simulink model "bpsk_transmitter"  (R2020a)
settings: Solver=VariableStepAuto  StartTime=0.0  StopTime=200/100e3  RelTol=1e-3
PreLoadFcn:
  | setup_bpsk_transmitter
InitFcn:
  | setup_bpsk_transmitter
undefined symbols (not defined in the file): AXI4, Lite, tx_data, xlfda_numerator
libraries: xbsIndex_r4 x43, hdlsllib x4, simulink x1
settings Model: Creator=David Northcote  LastModifiedBy=david
settings SFSimCC: CustomCodeUndefinedFunction=UseInterfaceOnly

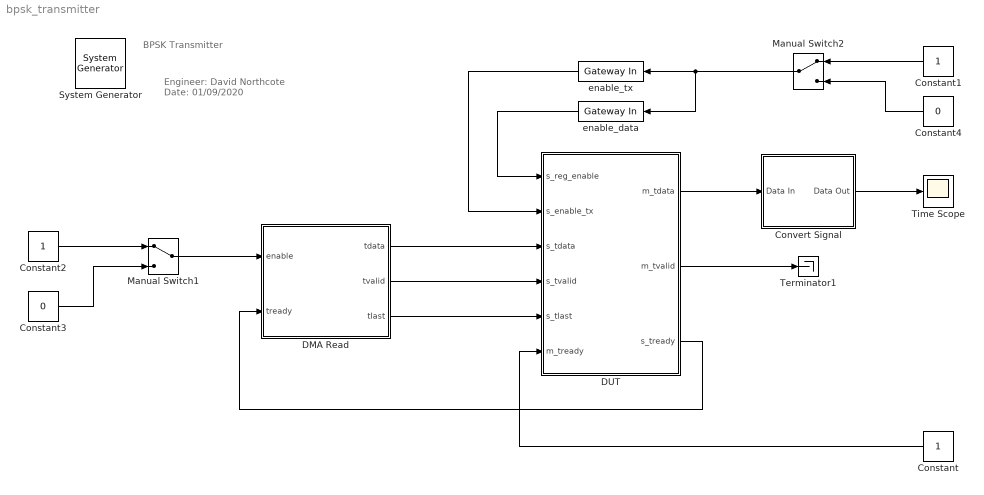
== system bpsk_transmitter ==
  note: Engineer:	David Northcote
      | Date:		01/09/2020
  note: BPSK Transmitter
  " System Generator" : xbsIndex_r4/ System Generator  Tag=genX  xilinxfamily=zynquplusRFSOC  part=xczu28dr  speed=-2-e  package=ffvg1517  synthesis_tool=Vivado  clock_wrapper=Clock Enables  directory=./netlist  proj_type=Vivado  Synth_file=Vivado Synthesis Defaults  Impl_file=Vivado Implementation Defaults  testbench=off  simulink_period=1/128e6  sysclk_period=(1/128e6)*1e9  dcm_input_clock_period=10  incr_netlist=off  trim_vbits=Everywhere in SubSystem  dbl_ovrd=According to Block Masks  core_generation=According to Block Masks  run_coregen=off  deprecated_control=off  eval_field=0  block_type=sysgen
  Constant : Constant  SampleTime=1/128e6
  Constant1 : Constant  OutDataTypeStr=boolean  SampleTime=1/(100e3)
  Constant2 : Constant  OutDataTypeStr=boolean  SampleTime=1/128e6
  Constant3 : Constant  Value=0  OutDataTypeStr=boolean  SampleTime=1/128e6
  Constant4 : Constant  Value=0  OutDataTypeStr=boolean  SampleTime=1/(100e3)
  Convert Signal : Subsystem
  DMA Read : Subsystem
  DUT : Subsystem
  Manual Switch1 : ManualSwitch
  Manual Switch2 : ManualSwitch
  Terminator1 : Terminator
  Time Scope : Scope
  enable_data : xbsIndex_r4/Gateway In  gui_display_data_type=Boolean  arith_type=Boolean  n_bits=16  bin_pt=14  preci_type=Single  exp_width=8  frac_width=24  rows=1  columns=1  quantization="Round  (unbiased: +/- Inf)"  overflow=Saturate  period=1/(100e3)  UseAsADC=off  ADCChannel='1'  interface=AXI4-Lite  automatic_assignment=off  address_offset=0  intf_name=''  intf_description=''  default_value=0  timing_constraint=None  locs_specified=off  LOCs={}  io_standard={}  inherit_from_input=off  hdl_port=on  dbl_ovrd=off  block_type=gatewayin
  enable_tx : xbsIndex_r4/Gateway In  gui_display_data_type=Boolean  arith_type=Boolean  n_bits=16  bin_pt=14  preci_type=Single  exp_width=8  frac_width=24  rows=1  columns=1  quantization="Round  (unbiased: +/- Inf)"  overflow=Saturate  period=1/(100e3)  UseAsADC=off  ADCChannel='1'  interface=AXI4-Lite  automatic_assignment=off  address_offset=4  intf_name=''  intf_description=''  default_value=0  timing_constraint=None  locs_specified=off  LOCs={}  io_standard={}  inherit_from_input=off  hdl_port=on  dbl_ovrd=off  block_type=gatewayin
  wires:
  Constant2/1 -> Manual Switch1/1
  Constant3/1 -> Manual Switch1/2
  Manual Switch1/1 -> DMA Read/1(enable)
  DMA Read/1(tdata) -> DUT/3(s_tdata)
  DMA Read/2(tvalid) -> DUT/4(s_tvalid)
  DMA Read/3(tlast) -> DUT/5(s_tlast)
  DUT/3(s_tready) -> DMA Read/2(tready)
  DUT/2(m_tvalid) -> Terminator1/1
  Constant/1 -> DUT/6(m_tready)
  enable_data/1 -> DUT/1(s_reg_enable)
  Constant4/1 -> Manual Switch2/2
  Constant1/1 -> Manual Switch2/1
  enable_tx/1 -> DUT/2(s_enable_tx)
  Manual Switch2/1 -> enable_data/1, enable_tx/1
  DUT/1(m_tdata) -> Convert Signal/1(Data In)
  Convert Signal/1(Data Out) -> Time Scope/1

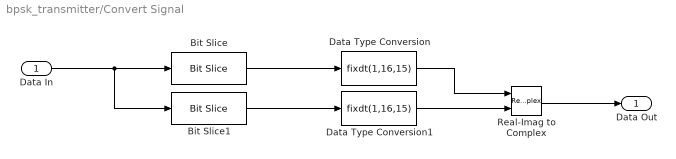
== system bpsk_transmitter/Convert Signal ==
  Data In : Inport
  Bit Slice : hdlsllib/Logic and Bit Operations/Bit Slice  lidx=15  ridx=0
      settings: SourceProductBaseCode=SL
  Bit Slice1 : hdlsllib/Logic and Bit Operations/Bit Slice  lidx=31  ridx=16
      settings: SourceProductBaseCode=SL
  Data Type Conversion : DataTypeConversion  OutDataTypeStr=fixdt(1,16,15)  ConvertRealWorld=Stored Integer (SI)
  Data Type Conversion1 : DataTypeConversion  OutDataTypeStr=fixdt(1,16,15)  ConvertRealWorld=Stored Integer (SI)
  Real-Imag to Complex : RealImagToComplex
  Data Out : Outport  VectorParamsAs1DForOutWhenUnconnected=off
  wires:
  Data Type Conversion1/1 -> Real-Imag to Complex/2
  Bit Slice/1 -> Data Type Conversion/1
  Data Type Conversion/1 -> Real-Imag to Complex/1
  Real-Imag to Complex/1 -> Data Out/1
  Data In/1 -> Bit Slice1/1, Bit Slice/1
  Bit Slice1/1 -> Data Type Conversion1/1

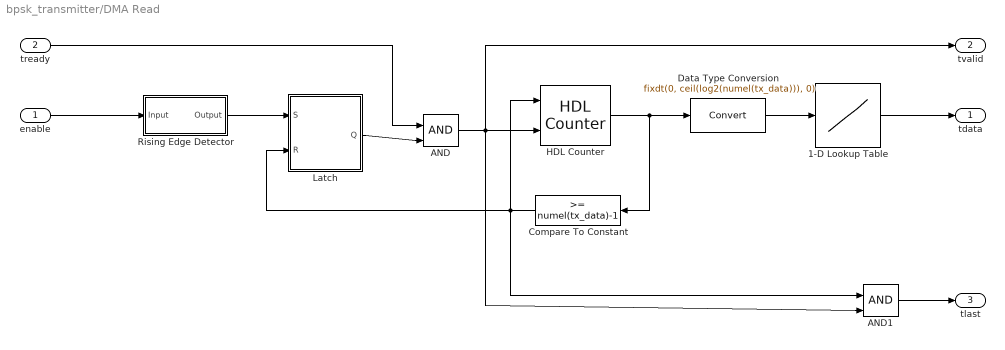
== system bpsk_transmitter/DMA Read ==
  enable : Inport
  tready : Inport  Port=2
  1-D Lookup Table : Lookup_n-D  NumberOfTableDimensions=1  BreakpointsForDimension1=[0:1:numel(tx_data)-1]  Table=tx_data  TableDataTypeStr=Inherit: Inherit from 'Table data'  ExtrapMethod=Clip  InternalRulePriority=Speed  OutDataTypeStr=Inherit: Inherit from 'Table data'  RndMeth=Simplest  InputSameDT=on
  AND : Logic  IconShape=distinctive  AllPortsSameDT=off  OutDataTypeStr=boolean
  AND1 : Logic  IconShape=distinctive  AllPortsSameDT=off  OutDataTypeStr=boolean
  Compare To Constant : simulink/Logic and Bit Operations/Compare To Constant  relop=>=  const=numel(tx_data)-1  OutDataTypeStr=boolean
  Data Type Conversion : DataTypeConversion  OutDataTypeStr=fixdt(0, ceil(log2(numel(tx_data))), 0)
  HDL Counter : hdlsllib/Sources/HDL Counter  CountType=Free running  CountInit=0  CountStep=1  CountMax=25  CountFromType=Initial value  CountFrom=0  CountResetPort=on  CountLoadPort=off  CountEnbPort=on  CountDirPort=off  CountDataType=Unsigned  CountWordLen=32  CountFracLen=0  CountSampTime=1
  Latch : Subsystem
  Rising Edge Detector : Subsystem
  tdata : Outport  VectorParamsAs1DForOutWhenUnconnected=off
  tvalid : Outport  Port=2  VectorParamsAs1DForOutWhenUnconnected=off
  tlast : Outport  Port=3  VectorParamsAs1DForOutWhenUnconnected=off
  wires:
  1-D Lookup Table/1 -> tdata/1
  Compare To Constant/1 -> AND1/1, HDL Counter/1, Latch/2(R)
  enable/1 -> Rising Edge Detector/1(Input)
  HDL Counter/1 -> Compare To Constant/1, Data Type Conversion/1
  Data Type Conversion/1 -> 1-D Lookup Table/1
  Rising Edge Detector/1(Output) -> Latch/1(S)
  AND/1 -> AND1/2, tvalid/1, HDL Counter/2
  Latch/1(Q) -> AND/2
  tready/1 -> AND/1
  AND1/1 -> tlast/1

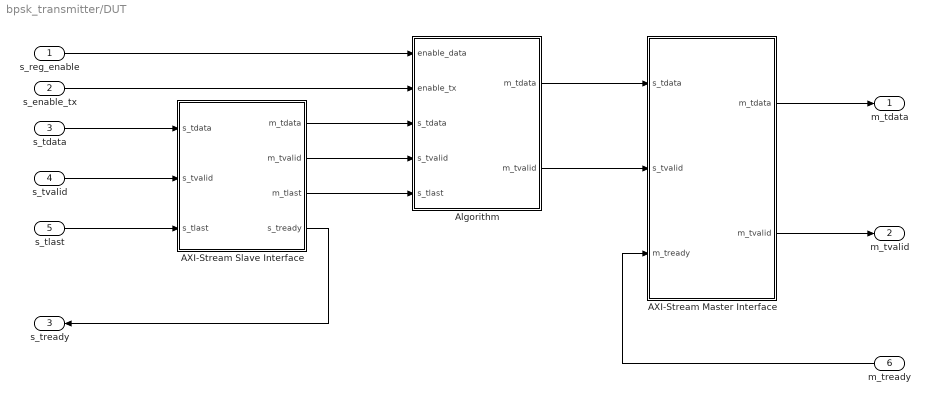
== system bpsk_transmitter/DUT ==
  s_reg_enable : Inport
  s_enable_tx : Inport  Port=2
  s_tdata : Inport  Port=3
  s_tvalid : Inport  Port=4
  s_tlast : Inport  Port=5
  m_tready : Inport  Port=6
  AXI-Stream Master Interface : Subsystem
  AXI-Stream Slave Interface : Subsystem
  Algorithm : Subsystem
  m_tdata : Outport  VectorParamsAs1DForOutWhenUnconnected=off
  m_tvalid : Outport  Port=2  VectorParamsAs1DForOutWhenUnconnected=off
  s_tready : Outport  Port=3  VectorParamsAs1DForOutWhenUnconnected=off
  wires:
  AXI-Stream Slave Interface/1(m_tdata) -> Algorithm/3(s_tdata)
  AXI-Stream Slave Interface/4(s_tready) -> s_tready/1
  AXI-Stream Master Interface/2(m_tvalid) -> m_tvalid/1
  AXI-Stream Slave Interface/2(m_tvalid) -> Algorithm/4(s_tvalid)
  AXI-Stream Slave Interface/3(m_tlast) -> Algorithm/5(s_tlast)
  Algorithm/1(m_tdata) -> AXI-Stream Master Interface/1(s_tdata)
  s_tvalid/1 -> AXI-Stream Slave Interface/2(s_tvalid)
  Algorithm/2(m_tvalid) -> AXI-Stream Master Interface/2(s_tvalid)
  AXI-Stream Master Interface/1(m_tdata) -> m_tdata/1
  m_tready/1 -> AXI-Stream Master Interface/3(m_tready)
  s_tdata/1 -> AXI-Stream Slave Interface/1(s_tdata)
  s_tlast/1 -> AXI-Stream Slave Interface/3(s_tlast)
  s_reg_enable/1 -> Algorithm/1(enable_data)
  s_enable_tx/1 -> Algorithm/2(enable_tx)

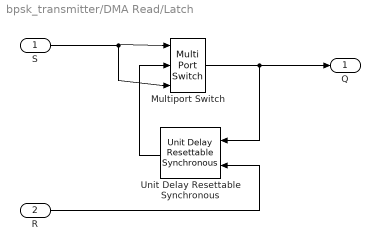
== system bpsk_transmitter/DMA Read/Latch ==
  S : Inport
  R : Inport  Port=2
  Multiport Switch : MultiPortSwitch  DataPortOrder=Zero-based contiguous  Inputs=2  zeroidx=on
  Unit Delay Resettable Synchronous : hdlsllib/Discrete/Unit Delay Resettable Synchronous  InitialCondition=0.0  SampleTime=-1
      settings: SourceProductBaseCode=SL
  Q : Outport  VectorParamsAs1DForOutWhenUnconnected=off
  wires:
  Multiport Switch/1 -> Unit Delay Resettable Synchronous/1, Q/1
  S/1 -> Multiport Switch/3, Multiport Switch/1
  Unit Delay Resettable Synchronous/1 -> Multiport Switch/2
  R/1 -> Unit Delay Resettable Synchronous/2

== system bpsk_transmitter/DMA Read/Rising Edge Detector ==
  Input : Inport
  AND1 : Logic  IconShape=distinctive  AllPortsSameDT=off  OutDataTypeStr=boolean
  Delay1 : Delay  DelayLength=1
  NOT : Logic  Operator=NOT  IconShape=distinctive  AllPortsSameDT=off  OutDataTypeStr=boolean
  Output : Outport  VectorParamsAs1DForOutWhenUnconnected=off
  wires:
  NOT/1 -> AND1/1
  Input/1 -> AND1/2, Delay1/1
  Delay1/1 -> NOT/1
  AND1/1 -> Output/1

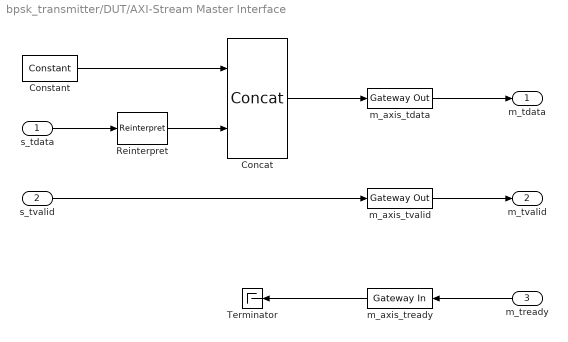
== system bpsk_transmitter/DUT/AXI-Stream Master Interface ==
  s_tdata : Inport
  s_tvalid : Inport  Port=2
  m_tready : Inport  Port=3
  Concat : xbsIndex_r4/Concat  num_inputs=2  dbl_ovrd=off  block_type=concat
  Constant : xbsIndex_r4/Constant  const=0  gui_display_data_type=Fixed-point  arith_type=Unsigned  n_bits=16  bin_pt=0  preci_type=Single  exp_width=8  frac_width=24  explicit_period=off  period=1  equ=P=C  opselect=C  inp2=PCIN>>17  opr=+  inp1=P  carry=CIN  dbl_ovrd=off  block_type=constant
  Reinterpret : xbsIndex_r4/Reinterpret  force_arith_type=on  arith_type=Unsigned  force_bin_pt=on  bin_pt=0  block_type=reinterpret
  Terminator : Terminator
  m_axis_tdata : xbsIndex_r4/Gateway Out  inherit_from_input=on  hdl_port=on  rows=1  columns=1  UseAsDAC=off  DACChannel='1'  interface=None  automatic_assignment=on  address_offset=hex2dec('00')  intf_name=''  intf_description=''  timing_constraint=None  locs_specified=off  LOCs={}  io_standard={}  block_type=gatewayout
  m_axis_tready : xbsIndex_r4/Gateway In  gui_display_data_type=Boolean  arith_type=Boolean  n_bits=16  bin_pt=14  preci_type=Single  exp_width=8  frac_width=24  rows=1  columns=1  quantization="Round  (unbiased: +/- Inf)"  overflow=Saturate  period=1/128e6  UseAsADC=off  ADCChannel='1'  interface=None  automatic_assignment=on  address_offset=hex2dec('00')  intf_name=''  intf_description=''  default_value=0  timing_constraint=None  locs_specified=off  LOCs={}  io_standard={}  inherit_from_input=off  hdl_port=on  dbl_ovrd=off  block_type=gatewayin
  m_axis_tvalid : xbsIndex_r4/Gateway Out  inherit_from_input=on  hdl_port=on  rows=1  columns=1  UseAsDAC=off  DACChannel='1'  interface=None  automatic_assignment=on  address_offset=hex2dec('00')  intf_name=''  intf_description=''  timing_constraint=None  locs_specified=off  LOCs={}  io_standard={}  block_type=gatewayout
  m_tdata : Outport  VectorParamsAs1DForOutWhenUnconnected=off
  m_tvalid : Outport  Port=2  VectorParamsAs1DForOutWhenUnconnected=off
  wires:
  m_axis_tvalid/1 -> m_tvalid/1
  s_tvalid/1 -> m_axis_tvalid/1
  m_axis_tdata/1 -> m_tdata/1
  m_tready/1 -> m_axis_tready/1
  m_axis_tready/1 -> Terminator/1
  Concat/1 -> m_axis_tdata/1
  s_tdata/1 -> Reinterpret/1
  Reinterpret/1 -> Concat/2
  Constant/1 -> Concat/1

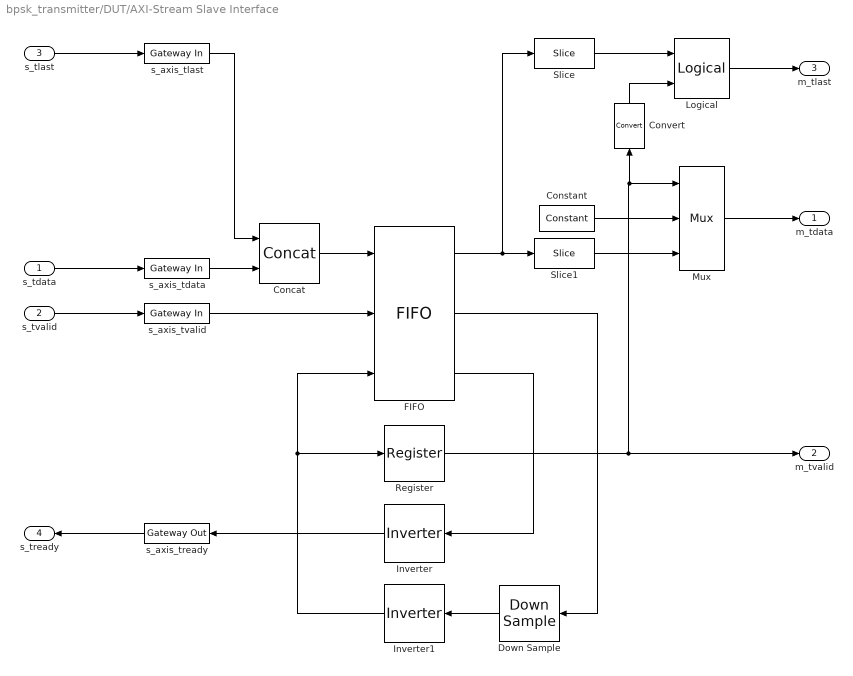
== system bpsk_transmitter/DUT/AXI-Stream Slave Interface ==
  s_tdata : Inport
  s_tvalid : Inport  Port=2
  s_tlast : Inport  Port=3
  Concat : xbsIndex_r4/Concat  num_inputs=2  dbl_ovrd=off  block_type=concat
  Constant : xbsIndex_r4/Constant  const=0  gui_display_data_type=Fixed-point  arith_type=Unsigned  n_bits=8  bin_pt=0  preci_type=Single  exp_width=8  frac_width=24  explicit_period=off  period=1  equ=P=C  opselect=C  inp2=PCIN>>17  opr=+  inp1=P  carry=CIN  dbl_ovrd=off  block_type=constant
  Convert : xbsIndex_r4/Convert  gui_display_data_type=Fixed-point  arith_type=Unsigned  n_bits=1  bin_pt=0  float_type=Single  exp_bits=8  fraction_bits=24  quantization=Truncate  overflow=Wrap  en=off  latency=0  pipeline=off  dbl_ovrd=off  block_type=convert
  Down Sample : xbsIndex_r4/Down Sample  sample_ratio=128e6/12.5e3  sample_phase=First Value of Frame  en=off  rst=off  latency=0  dbl_ovrd=off  block_type=dsamp
  FIFO : xbsIndex_r4/FIFO  mem_type=Block RAM  performance_options=Standard_FIFO  embedded_registers=off  depth=1K  percent_nbits=2  rst=off  rst_latency=2  en=off  use_dcount=off  use_percent_full_port=off  use_almost_empty=off  almost_empty_thresh=2  use_almost_full=off  use_rd_rst_busy=off  use_wr_rst_busy=off  almost_full_thresh=1000  explicit_period=off  dbl_ovrd=off  simulation_type=fast_sim  block_type=fifo
  Inverter : xbsIndex_r4/Inverter  en=off  latency=0  dbl_ovrd=off  block_type=inv
  Inverter1 : xbsIndex_r4/Inverter  en=off  latency=0  dbl_ovrd=off  block_type=inv
  Logical : xbsIndex_r4/Logical  logical_function=AND  inputs=2  en=off  latency=0  precision=Full  arith_type=Unsigned  n_bits=16  bin_pt=0  align_bp=on  dbl_ovrd=off  block_type=logical
  Mux : xbsIndex_r4/Mux  inputs=2  en=off  latency=0  precision=Full  arith_type=Unsigned  n_bits=16  bin_pt=14  quantization=Truncate  overflow=Wrap  dbl_ovrd=off  block_type=mux
  Register : xbsIndex_r4/Register  init=0  rst=off  en=off  dbl_ovrd=off  block_type=register
  Slice : xbsIndex_r4/Slice  nbits=1  boolean_output=off  mode=Two Bit Locations  bit1=8  base1=LSB of Input  bit0=8  base0=LSB of Input  dbl_ovrd=off  block_type=slice
  Slice1 : xbsIndex_r4/Slice  nbits=1  boolean_output=off  mode=Two Bit Locations  bit1=7  base1=LSB of Input  bit0=0  base0=LSB of Input  dbl_ovrd=off  block_type=slice
  s_axis_tdata : xbsIndex_r4/Gateway In  gui_display_data_type=Fixed-point  arith_type=Unsigned  n_bits=8  bin_pt=0  preci_type=Single  exp_width=8  frac_width=24  rows=1  columns=1  quantization="Round  (unbiased: +/- Inf)"  overflow=Saturate  period=1/128e6  UseAsADC=off  ADCChannel='1'  interface=None  automatic_assignment=on  address_offset=hex2dec('00')  intf_name=''  intf_description=''  default_value=0  timing_constraint=None  locs_specified=off  LOCs={}  io_standard={}  inherit_from_input=off  hdl_port=on  dbl_ovrd=off  block_type=gatewayin
  s_axis_tlast : xbsIndex_r4/Gateway In  gui_display_data_type=Fixed-point  arith_type=Unsigned  n_bits=1  bin_pt=0  preci_type=Single  exp_width=8  frac_width=24  rows=1  columns=1  quantization="Round  (unbiased: +/- Inf)"  overflow=Saturate  period=1/128e6  UseAsADC=off  ADCChannel='1'  interface=None  automatic_assignment=on  address_offset=hex2dec('00')  intf_name=''  intf_description=''  default_value=0  timing_constraint=None  locs_specified=off  LOCs={}  io_standard={}  inherit_from_input=off  hdl_port=on  dbl_ovrd=off  block_type=gatewayin
  s_axis_tready : xbsIndex_r4/Gateway Out  inherit_from_input=on  hdl_port=on  rows=1  columns=1  UseAsDAC=off  DACChannel='1'  interface=None  automatic_assignment=on  address_offset=hex2dec('00')  intf_name=''  intf_description=''  timing_constraint=None  locs_specified=off  LOCs={}  io_standard={}  block_type=gatewayout
  s_axis_tvalid : xbsIndex_r4/Gateway In  gui_display_data_type=Boolean  arith_type=Boolean  n_bits=16  bin_pt=14  preci_type=Single  exp_width=8  frac_width=24  rows=1  columns=1  quantization="Round  (unbiased: +/- Inf)"  overflow=Saturate  period=1/128e6  UseAsADC=off  ADCChannel='1'  interface=None  automatic_assignment=on  address_offset=hex2dec('00')  intf_name=''  intf_description=''  default_value=0  timing_constraint=None  locs_specified=off  LOCs={}  io_standard={}  inherit_from_input=off  hdl_port=on  dbl_ovrd=off  block_type=gatewayin
  m_tdata : Outport  VectorParamsAs1DForOutWhenUnconnected=off
  m_tvalid : Outport  Port=2  VectorParamsAs1DForOutWhenUnconnected=off
  m_tlast : Outport  Port=3  VectorParamsAs1DForOutWhenUnconnected=off
  s_tready : Outport  Port=4  VectorParamsAs1DForOutWhenUnconnected=off
  wires:
  s_axis_tready/1 -> s_tready/1
  s_tlast/1 -> s_axis_tlast/1
  s_tvalid/1 -> s_axis_tvalid/1
  s_tdata/1 -> s_axis_tdata/1
  s_axis_tvalid/1 -> FIFO/2
  FIFO/3 -> Inverter/1
  Down Sample/1 -> Inverter1/1
  FIFO/2 -> Down Sample/1
  Register/1 -> Mux/1, Convert/1, m_tvalid/1
  Inverter/1 -> s_axis_tready/1
  Inverter1/1 -> Register/1, FIFO/3
  Logical/1 -> m_tlast/1
  Mux/1 -> m_tdata/1
  FIFO/1 -> Slice/1, Slice1/1
  Constant/1 -> Mux/2
  Convert/1 -> Logical/2
  Slice/1 -> Logical/1
  Concat/1 -> FIFO/1
  s_axis_tdata/1 -> Concat/2
  s_axis_tlast/1 -> Concat/1
  Slice1/1 -> Mux/3

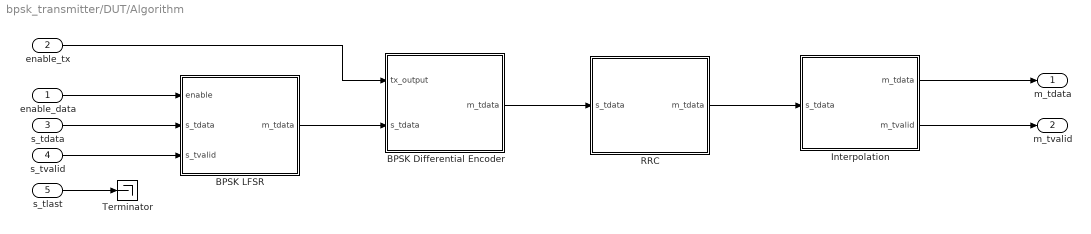
== system bpsk_transmitter/DUT/Algorithm ==
  enable_data : Inport
  enable_tx : Inport  Port=2
  s_tdata : Inport  Port=3
  s_tvalid : Inport  Port=4
  s_tlast : Inport  Port=5
  BPSK Differential Encoder : Subsystem
  BPSK LFSR : Subsystem
  Interpolation : Subsystem
  RRC : Subsystem
  Terminator : Terminator
  m_tdata : Outport  VectorParamsAs1DForOutWhenUnconnected=off
  m_tvalid : Outport  Port=2  VectorParamsAs1DForOutWhenUnconnected=off
  wires:
  BPSK LFSR/1(m_tdata) -> BPSK Differential Encoder/2(s_tdata)
  BPSK Differential Encoder/1(m_tdata) -> RRC/1(s_tdata)
  s_tlast/1 -> Terminator/1
  s_tdata/1 -> BPSK LFSR/2(s_tdata)
  s_tvalid/1 -> BPSK LFSR/3(s_tvalid)
  enable_data/1 -> BPSK LFSR/1(enable)
  RRC/1(m_tdata) -> Interpolation/1(s_tdata)
  Interpolation/2(m_tvalid) -> m_tvalid/1
  Interpolation/1(m_tdata) -> m_tdata/1
  enable_tx/1 -> BPSK Differential Encoder/1(tx_output)

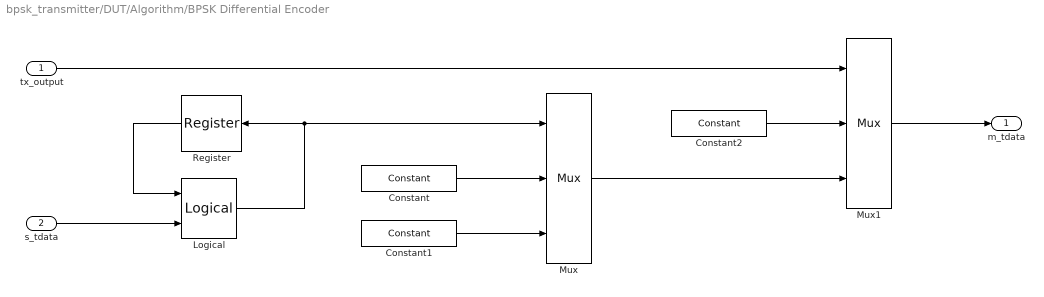
== system bpsk_transmitter/DUT/Algorithm/BPSK Differential Encoder ==
  tx_output : Inport
  s_tdata : Inport  Port=2
  Constant : xbsIndex_r4/Constant  const=1/sqrt(2)  gui_display_data_type=Fixed-point  arith_type=Signed (2's comp)  n_bits=16  bin_pt=15  preci_type=Single  exp_width=8  frac_width=24  explicit_period=off  period=1  equ=P=C  opselect=C  inp2=PCIN>>17  opr=+  inp1=P  carry=CIN  dbl_ovrd=off  block_type=constant
  Constant1 : xbsIndex_r4/Constant  const=-1/sqrt(2)  gui_display_data_type=Fixed-point  arith_type=Signed (2's comp)  n_bits=16  bin_pt=15  preci_type=Single  exp_width=8  frac_width=24  explicit_period=off  period=1  equ=P=C  opselect=C  inp2=PCIN>>17  opr=+  inp1=P  carry=CIN  dbl_ovrd=off  block_type=constant
  Constant2 : xbsIndex_r4/Constant  const=0  gui_display_data_type=Fixed-point  arith_type=Signed (2's comp)  n_bits=16  bin_pt=15  preci_type=Single  exp_width=8  frac_width=24  explicit_period=off  period=1  equ=P=C  opselect=C  inp2=PCIN>>17  opr=+  inp1=P  carry=CIN  dbl_ovrd=off  block_type=constant
  Logical : xbsIndex_r4/Logical  logical_function=XOR  inputs=2  en=off  latency=0  precision=Full  arith_type=Unsigned  n_bits=16  bin_pt=0  align_bp=on  dbl_ovrd=off  block_type=logical
  Mux : xbsIndex_r4/Mux  inputs=2  en=off  latency=1  precision=Full  arith_type=Unsigned  n_bits=16  bin_pt=14  quantization=Truncate  overflow=Wrap  dbl_ovrd=off  block_type=mux
  Mux1 : xbsIndex_r4/Mux  inputs=2  en=off  latency=1  precision=Full  arith_type=Unsigned  n_bits=16  bin_pt=14  quantization=Truncate  overflow=Wrap  dbl_ovrd=off  block_type=mux
  Register : xbsIndex_r4/Register  init=0  rst=off  en=off  dbl_ovrd=off  block_type=register
  m_tdata : Outport  VectorParamsAs1DForOutWhenUnconnected=off
  wires:
  Logical/1 -> Register/1, Mux/1
  Register/1 -> Logical/1
  s_tdata/1 -> Logical/2
  Constant/1 -> Mux/2
  Constant1/1 -> Mux/3
  Mux/1 -> Mux1/3
  Mux1/1 -> m_tdata/1
  Constant2/1 -> Mux1/2
  tx_output/1 -> Mux1/1

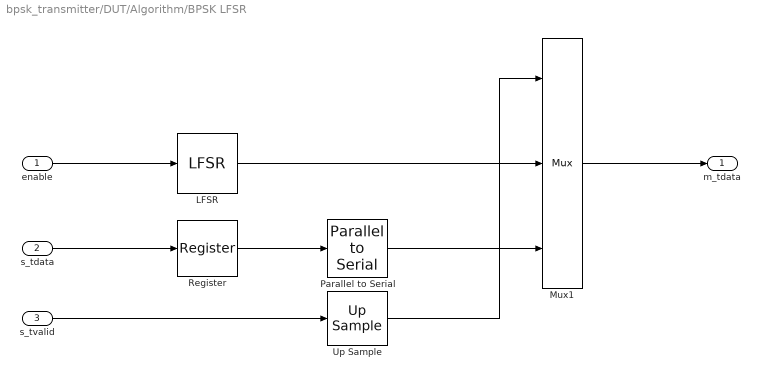
== system bpsk_transmitter/DUT/Algorithm/BPSK LFSR ==
  enable : Inport
  s_tdata : Inport  Port=2
  s_tvalid : Inport  Port=3
  LFSR : xbsIndex_r4/LFSR  lfsr_type=Fibonacci  gate_type=XNOR  n_bits=10  maxpolynomial=on  polynomial='121'  rst_value='011'  rst=off  en=on  reloadable_seed=off  input_type=off  output_type=off  arith_type="Signed  (2's comp)"  bin_pt=4  explicit_period=off  period=1  dbl_ovrd=off  block_type=lfsr
  Mux1 : xbsIndex_r4/Mux  inputs=2  en=off  latency=0  precision=Full  arith_type=Unsigned  n_bits=16  bin_pt=14  quantization=Truncate  overflow=Wrap  dbl_ovrd=off  block_type=mux
  Parallel to Serial : xbsIndex_r4/Parallel to Serial  output_order=Least Significant Word First  arith_type=Unsigned  output_bits=1  bin_pt=0  rst=off  en=off  latency=0  dbl_ovrd=off  block_type=p2s
      settings: infoedit=Each sample presented at the input becomes several samples presented serially at the output.
  Register : xbsIndex_r4/Register  init=0  rst=off  en=off  dbl_ovrd=off  block_type=register
  Up Sample : xbsIndex_r4/Up Sample  sample_ratio=8  copy_samples=on  en=off  latency=1  dbl_ovrd=off  block_type=usamp
  m_tdata : Outport  VectorParamsAs1DForOutWhenUnconnected=off
  wires:
  Register/1 -> Parallel to Serial/1
  Parallel to Serial/1 -> Mux1/3
  s_tdata/1 -> Register/1
  s_tvalid/1 -> Up Sample/1
  Up Sample/1 -> Mux1/1
  enable/1 -> LFSR/1
  Mux1/1 -> m_tdata/1
  LFSR/1 -> Mux1/2

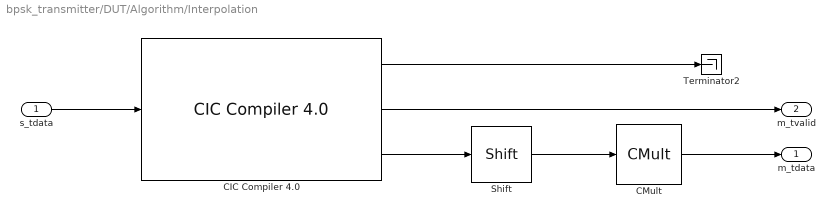
== system bpsk_transmitter/DUT/Algorithm/Interpolation ==
  s_tdata : Inport
  "CIC Compiler 4.0 " : xbsIndex_r4/CIC Compiler 4.0   filter_type=Interpolation  number_of_stages=5  differential_delay=1  number_of_channels=1  sample_rate_changes=Fixed  fixed_or_initial_rate=128e6/400e3  minimum_rate=320  maximum_rate=320  ratespecification=Maximum_Possible  sampleperiod=320  hardwareoversamplingrate=1  quantization=Full_Precision  output_data_width=52  use_xtreme_dsp_slice=on  use_streaming_interface=on  has_aclken=off  has_aresetn=off  has_dout_tready=off  trim_axipin_name=on  gui_behaviour=Sysgen_GUI  input_data_width=18  ip_name=CIC Compiler  ip_version=4.0  dsptool_ready=true  wrapper_available=true  port_translation_map={ 'aclken' => 'en', 'aresetn' => 'rst' }  ipcore_xco_need_fpga_part=true  ipcore_verbose=false  block_type=cic_compiler_v4_0
  CMult : xbsIndex_r4/CMult  const=1/((((128e6/400e3)^5)/(128e6/400e3))*2^-33)  gui_display_data_type=Fixed-point  const_n_bits=16  const_bin_pt=15  float_type=Single  exp_bits=8  fraction_bits=24  en=off  latency=1  precision=User Defined  arith_type="Signed  (2's comp)"  n_bits=16  bin_pt=15  quantization="Round  (unbiased: +/- Inf)"  overflow=Saturate  use_behavioral_HDL=off  mem_type=Distributed RAM  pipeline=off  dbl_ovrd=off  block_type=cmult
  Shift : xbsIndex_r4/Shift  shift_dir=Right  shift_bits=floor(log2(((128e6/400e3)^5)/(128e6/400e3)))  en=off  latency=0  precision=User Defined  arith_type="Signed  (2's comp)"  n_bits=ceil(log2(((128e6/100e3)^5)/(128e6/100e3)))+16  bin_pt=ceil(log2(((128e6/100e3)^5)/(128e6/100e3)))+16-2  quantization="Round  (unbiased: +/- Inf)"  overflow=Saturate  dbl_ovrd=off  block_type=shift
  Terminator2 : Terminator
  m_tdata : Outport  VectorParamsAs1DForOutWhenUnconnected=off
  m_tvalid : Outport  Port=2  VectorParamsAs1DForOutWhenUnconnected=off
  wires:
  "CIC Compiler 4.0 "/2 -> m_tvalid/1
  "CIC Compiler 4.0 "/3 -> Shift/1
  "CIC Compiler 4.0 "/1 -> Terminator2/1
  Shift/1 -> CMult/1
  s_tdata/1 -> "CIC Compiler 4.0 "/1
  CMult/1 -> m_tdata/1

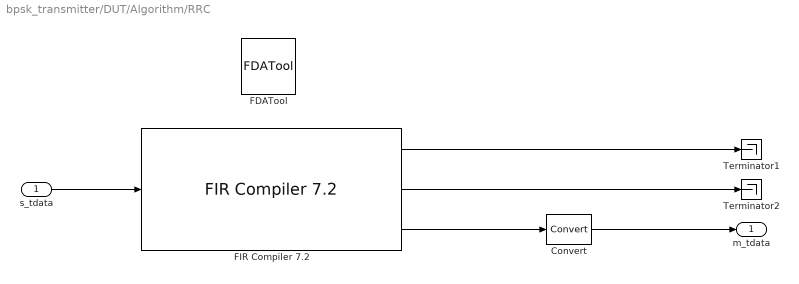
== system bpsk_transmitter/DUT/Algorithm/RRC ==
  s_tdata : Inport
  Convert : xbsIndex_r4/Convert  gui_display_data_type=Fixed-point  arith_type="Signed  (2's comp)"  n_bits=16  bin_pt=15  float_type=Single  exp_bits=8  fraction_bits=24  quantization="Round  (unbiased: +/- Inf)"  overflow=Saturate  en=off  latency=0  pipeline=off  dbl_ovrd=off  block_type=convert
  FDATool : xbsIndex_r4/FDATool  block_type=fdatool
      settings: infoedit=FDATool
  "FIR Compiler 7.2 " : xbsIndex_r4/FIR Compiler 7.2   coefficientvector=xlfda_numerator('FDATool')*4  coefficient_sets=1  coefficient_reload=off  filter_type=Interpolation  rate_change_type=Integer  interpolation_rate=4  decimation_rate=1  zero_pack_factor=1  channel_sequence=Basic  number_channels=1  pattern_list='P4-0,P4-1,P4-2,P4-3,P4-4'  number_paths=1  ratespecification=Maximum_Possible  sampleperiod=1280  hardwareoversamplingrate=1  coefficient_sign=Signed  quantization=Quantize_Only  coefficient_width=16  bestprecision=on  coefficient_fractional_bits=14  coefficient_structure=Inferred  output_rounding_mode=Full_Precision  output_width=31  filter_architecture=Systolic_Multiply_Accumulate  optimization_goal=Area  optimization_list='None'  data_buffer_type=Automatic  coefficient_buffer_type=Automatic  input_buffer_type=Automatic  output_buffer_type=Automatic  preference_for_other_storage=Automatic  multi_column_support=Automatic  columnconfig='6'  inter_column_pipe_length=4  data_has_tlast=Not_Required  m_data_has_tready=off  s_data_has_fifo=off  s_data_has_tuser=Not_Required  m_data_has_tuser=Not_Required  s_config_sync_mode=On_Vector  s_config_method=Single  num_reload_slots=1  has_aclken=off  has_aresetn=off  infoeditControl=ARESETn must be asserted for a minimum of 2 cycles  reset_data_vector=on  trim_axipin_name=on  simulation_type=hybrid_sim  simulation_model=sysgen:xfirv7_2_cmodel  data_path_portlist={ 's_axis_data_tdata', 'm_axis_data_tdata' }  passband_min=0.0  passband_max=0.5  stopband_min=0.5  stopband_max=1.0  filter_selection=1  gui_behaviour='Sysgen_GUI'  data_sign=Signed  data_width=16  data_fractional_bits=0  data_tuser_width=1  wrapper_available=true  ip_wrap_arbitrary_binary_point=true  ip_name=FIR Compiler  ip_version=7.2  dsptool_ready=true  ipcore_usecache=true  ipcore_useipmodelcache=true  port_translation_map={ 'aclken' => 'en', 'aresetn' => 'rst' }  run_core_at_system_period=true  ipcore_xco_need_fpga_part=true  block_type=fir_compiler_v7_2
      settings: infoedit=Maximum Possible : Maximizes oversampling rate. Abstracted input handshake (no s_data_tvalid) and automatic rate propagation.<br>Hardware Oversampling Rate : Specifies oversampling rate relative to the input sample period. Abstracted input handshake (no s_data_tvalid) and automatic rate propagation.<br>Input/Output Sample Period : Specifies absolute oversampling rate. No input handshake abstraction (exposes s_data_tvalid) and no rate propagation.
  Terminator1 : Terminator
  Terminator2 : Terminator
  m_tdata : Outport  VectorParamsAs1DForOutWhenUnconnected=off
  wires:
  s_tdata/1 -> "FIR Compiler 7.2 "/1
  "FIR Compiler 7.2 "/1 -> Terminator1/1
  Convert/1 -> m_tdata/1
  "FIR Compiler 7.2 "/3 -> Convert/1
  "FIR Compiler 7.2 "/2 -> Terminator2/1
